simulink model "MDOF_IP"  (R2023a)
settings: Solver=VariableStepAuto  StartTime=0.0  StopTime=window  FixedStep=SimStep  RelTol=1e-3
values from neighbouring files (symbols this model uses):
  SimStep = 0.01    [Part1_01_Geneartion_Configuration.m]
undefined symbols (not defined in the file or in its folder): Ai, Bi, Ci, Di, me
settings Model: Creator=cuishuaiwen  LastModifiedBy=cuishuaiwen
settings SolverCC: ZeroCrossAlgorithm=Adaptive
settings OptimizationCC: ReuseModelBlockBuffer=off

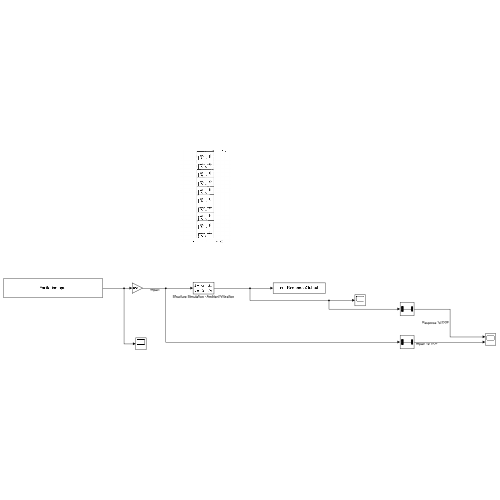
[thumbnail: Simulink's stored preview of the top-level diagram]
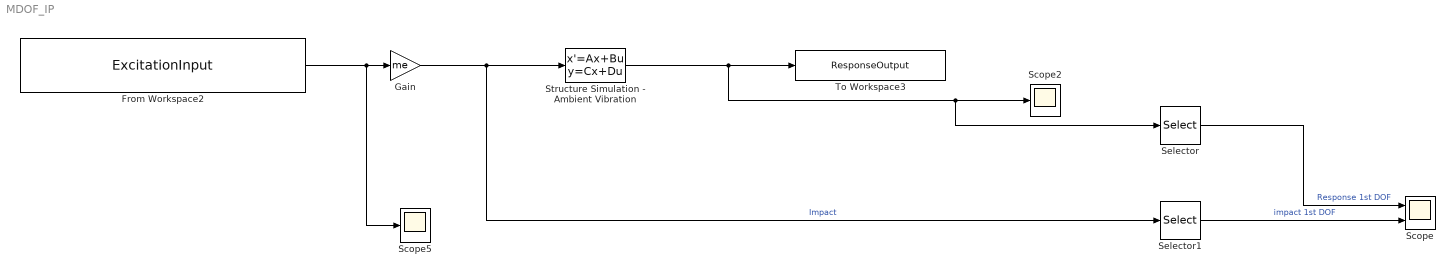
== system MDOF_IP ==
  From Workspace2 : FromWorkspace  VariableName=ExcitationInput  SampleTime=SimStep
  Gain : Gain  Gain=me
  Scope : Scope  NumInputPorts=2
  Scope2 : Scope
  Scope5 : Scope
  Selector : Selector  InputPortWidth=nDOF  IndexOptions=Index vector (dialog)  Indices=nDOF  OutputSizes=1
  Selector1 : Selector  InputPortWidth=nDOF  IndexOptions=Index vector (dialog)  Indices=nDOF  OutputSizes=1
  Structure Simulation - Ambient Vibration : StateSpace  A=Ai  B=Bi  C=Ci  D=Di  InitialCondition=0
  To Workspace3 : ToWorkspace  VariableName=ResponseOutput  SaveFormat=Structure With Time  SampleTime=SimStep
  wires:
  Structure Simulation - Ambient Vibration/1 -> Selector/1, Scope2/1, To Workspace3/1
  From Workspace2/1 -> Scope5/1, Gain/1
  Selector/1 -> Scope/1  "Response 1st DOF"
  Gain/1 -> Structure Simulation - Ambient Vibration/1, Selector1/1  "Impact"
  Selector1/1 -> Scope/2  "impact 1st DOF"
